simulink model "simulink_rosbag"  (R2020b)
settings: Solver=VariableStepAuto  StartTime=0.0  StopTime=inf  RelTol=1e-3
model workspace (MAT data in the model file):
  Logfile_Data_Object = robotics.ros.BagSelection
  Logfile_Data_Object.FilePath = 'C:\Users\ONLY-GOD\Documents\MATLAB\Examples\R2019b\rosbag\rosbagdata_1.bag'
  Logfile_Data_Object.StartTime = 1606974195.78
  Logfile_Data_Object.EndTime = 1606974582.7
  Logfile_Data_Object.NumMessages = 16443
  Logfile_Data_Object.AvailableTopics = table
  Logfile_Data_Object.AvailableTopics.data{1} = [966; 3865; 11607; 5]
  Logfile_Data_Object.AvailableTopics.data{2} = categorical
  Logfile_Data_Object.AvailableTopics.data{2}.categoryNames = {'nav_msgs/Odometry'; 'rosgraph_msgs/Log'; 'sensor_msgs/Imu'; 'sensor_msgs/NavSatFix'}
  Logfile_Data_Object.AvailableTopics.data{2}.codes = [4; 1; 3; 2]
  Logfile_Data_Object.AvailableTopics.data{3}{1} = '  uint32 Seq
    |   Time Stamp
    |   char FrameId
    | sensor_msgs/NavSatStatus Status
    |   int8 STATUSNOFIX
    |   int8 STATUSFIX
    |   int8 STATUSSBASFIX
    |   int8 STATUSGBASFIX
    |   int8 Status
    |   uint16 SERVICEGPS
    |   uint16 SERVICEGLONASS
    |   uint16 SERVICECOMPASS
    |   uint16 SERVICEGALILEO
    |   uint16 Service
    | double Latitude
    | double Longitude
    | double Altitude
    | double[9] PositionCovariance
    | uint8 COVARIANCETYPEUNKNOWN
    | uint8 COVARIANCETYPEAPPROXIMATED
    | uint8 COVARIANCETYPEDIAGONALKNOWN
    | uint8 COVARIANCETYPEKNOWN
    | uint8 PositionCovarianceType
    | '
  Logfile_Data_Object.AvailableTopics.data{3}{2} = '  uint32 Seq
    |   Time Stamp
    |   char FrameId
    | char ChildFrameId
    | geometry_msgs/PoseWithCovariance Pose
    |   geometry_msgs/Pose Pose
    |     geometry_msgs/Point Position
    |       double X
    |       double Y
    |       double Z
    |     geometry_msgs/Quaternion Orientation
    |       double X
    |       double Y
    |       double Z
    |       double W
    |   double[36] Covariance
    | geometry_msgs/TwistWithCovariance Twist
    |   geometry_msgs/Twist Twist
    |     geometry_msgs/Vector3 Linear
    |       double X
    |       double Y
    |       double Z
    |     geometry_msgs/Vector3 Angular
    |       double X
    |       double Y
    |       double Z
    |   double[36] Covariance
    | '
  Logfile_Data_Object.AvailableTopics.data{3}{3} = '  uint32 Seq
    |   Time Stamp
    |   char FrameId
    | geometry_msgs/Quaternion Orientation
    |   double X
    |   double Y
    |   double Z
    |   double W
    | double[9] OrientationCovariance
    | geometry_msgs/Vector3 AngularVelocity
    |   double X
    |   double Y
    |   double Z
    | double[9] AngularVelocityCovariance
    | geometry_msgs/Vector3 LinearAcceleration
    |   double X
    |   double Y
    |   double Z
    | double[9] LinearAccelerationCovariance
    | '
  Logfile_Data_Object.AvailableTopics.data{3}{4} = 'int8 INFO
    | int8 WARN
    | int8 ERROR
    | int8 FATAL
    | std_msgs/Header Header
    |   uint32 Seq
    |   Time Stamp
    |   char FrameId
    | int8 Level
    | char Name
    | char Msg
    | char File
    | char Function
    | uint32 Line
    | char[] Topics
    | '
  Logfile_Data_Object.AvailableTopics.ndims = 2
  Logfile_Data_Object.AvailableTopics.nrows = 4
  Logfile_Data_Object.AvailableTopics.rownames = {'/fix'; '/husky_velocity_controller/odom'; '/imu/data'; '/rosout'}
  Logfile_Data_Object.AvailableTopics.nvars = 3
  Logfile_Data_Object.AvailableTopics.varnames = {'NumMessages', 'MessageType', 'MessageDefinition'}
  Logfile_Data_Object.AvailableTopics.props.useVariableNamesOriginal = 0
  Logfile_Data_Object.AvailableTopics.props.useDimensionNamesOriginal = 0
  Logfile_Data_Object.AvailableTopics.props.CustomProps = struct()
  Logfile_Data_Object.AvailableTopics.props.VariableCustomProps = struct()
  Logfile_Data_Object.AvailableTopics.props.versionSavedFrom = 4
  Logfile_Data_Object.AvailableTopics.props.minCompatibleVersion = 1
  Logfile_Data_Object.AvailableTopics.props.incompatibilityMsg = ''
  Logfile_Data_Object.AvailableTopics.props.VersionSavedFrom = 4
  Logfile_Data_Object.AvailableTopics.props.Description = ''
  Logfile_Data_Object.AvailableTopics.props.VariableNamesOriginal = {}
  Logfile_Data_Object.AvailableTopics.props.DimensionNames = {'Row', 'Variables'}
  Logfile_Data_Object.AvailableTopics.props.DimensionNamesOriginal = {}
  Logfile_Data_Object.AvailableTopics.props.UserData = []
  Logfile_Data_Object.AvailableTopics.props.VariableDescriptions = {}
  Logfile_Data_Object.AvailableTopics.props.VariableUnits = {}
  Logfile_Data_Object.AvailableTopics.props.VariableContinuity = {}
  Logfile_Data_Object.MessageList = table
  Logfile_Data_Object.MessageList.data{1} = [1606974195.78 1606974195.78 1606974195.78 1606974195.78 1606974196 1606974196.09 1606974196.09 1606974196.09 1606974196.09 1606974196.12 1606974196.13 1606974196.16 ... (16443 elements, 16443x1)]
  Logfile_Data_Object.MessageList.data{2} = categorical
  Logfile_Data_Object.MessageList.data{2}.categoryNames = {'/fix'; '/husky_velocity_controller/odom'; '/imu/data'; '/rosout'}
  Logfile_Data_Object.MessageList.data{2}.codes = [4 4 4 4 4 3 3 2 3 3 2 3 ... (16443 elements, 16443x1)]
  Logfile_Data_Object.MessageList.data{3} = categorical
  Logfile_Data_Object.MessageList.data{3}.categoryNames = {'sensor_msgs/NavSatFix'; 'nav_msgs/Odometry'; 'sensor_msgs/Imu'; 'rosgraph_msgs/Log'}
  Logfile_Data_Object.MessageList.data{3}.codes = [4 4 4 4 4 3 3 2 3 3 2 3 ... (16443 elements, 16443x1)]
  Logfile_Data_Object.MessageList.data{4} = [5486 5746 6008 6272 7849 10576 10942 14932 11308 15691 16057 16816 ... (16443 elements, 16443x1)]
  Logfile_Data_Object.MessageList.ndims = 2
  Logfile_Data_Object.MessageList.nrows = 16443
  Logfile_Data_Object.MessageList.nvars = 4
  Logfile_Data_Object.MessageList.varnames = {'Time', 'Topic', 'MessageType', 'FileOffset'}
  Logfile_Data_Object.MessageList.props.useVariableNamesOriginal = 0
  Logfile_Data_Object.MessageList.props.useDimensionNamesOriginal = 0
  Logfile_Data_Object.MessageList.props.CustomProps = struct()
  Logfile_Data_Object.MessageList.props.VariableCustomProps = struct()
  Logfile_Data_Object.MessageList.props.versionSavedFrom = 4
  Logfile_Data_Object.MessageList.props.minCompatibleVersion = 1
  Logfile_Data_Object.MessageList.props.incompatibilityMsg = ''
  Logfile_Data_Object.MessageList.props.VersionSavedFrom = 4
  Logfile_Data_Object.MessageList.props.Description = ''
  Logfile_Data_Object.MessageList.props.VariableNamesOriginal = {}
  Logfile_Data_Object.MessageList.props.DimensionNames = {'Row', 'Variables'}
  Logfile_Data_Object.MessageList.props.DimensionNamesOriginal = {}
  Logfile_Data_Object.MessageList.props.UserData = []
  Logfile_Data_Object.MessageList.props.VariableDescriptions = {}
  Logfile_Data_Object.MessageList.props.VariableUnits = {}
  Logfile_Data_Object.MessageList.props.VariableContinuity = {}
  Logfile_Data_Object.TopicTypeMap = containers.Map
  Logfile_Data_Object.TopicTypeMap.serialization.keys = {'/fix', '/husky_velocity_controller/odom', '/imu/data', '/rosout'}
  Logfile_Data_Object.TopicTypeMap.serialization.values = {'sensor_msgs/NavSatFix', 'nav_msgs/Odometry', 'sensor_msgs/Imu', 'rosgraph_msgs/Log'}
  Logfile_Data_Object.TopicTypeMap.serialization.uniformity = 1
  Logfile_Data_Object.TopicTypeMap.serialization.keyType = 'char'
  Logfile_Data_Object.TopicTypeMap.serialization.valueType = 'char'
  Logfile_Data_Object.TopicDefinitionMap = containers.Map
  Logfile_Data_Object.TopicDefinitionMap.serialization.keys = {'/fix', '/husky_velocity_controller/odom', '/imu/data', '/rosout'}
  Logfile_Data_Object.TopicDefinitionMap.serialization.values{1} = '  uint32 Seq
    |   Time Stamp
    |   char FrameId
    | sensor_msgs/NavSatStatus Status
    |   int8 STATUSNOFIX
    |   int8 STATUSFIX
    |   int8 STATUSSBASFIX
    |   int8 STATUSGBASFIX
    |   int8 Status
    |   uint16 SERVICEGPS
    |   uint16 SERVICEGLONASS
    |   uint16 SERVICECOMPASS
    |   uint16 SERVICEGALILEO
    |   uint16 Service
    | double Latitude
    | double Longitude
    | double Altitude
    | double[9] PositionCovariance
    | uint8 COVARIANCETYPEUNKNOWN
    | uint8 COVARIANCETYPEAPPROXIMATED
    | uint8 COVARIANCETYPEDIAGONALKNOWN
    | uint8 COVARIANCETYPEKNOWN
    | uint8 PositionCovarianceType
    | '
  Logfile_Data_Object.TopicDefinitionMap.serialization.values{2} = '  uint32 Seq
    |   Time Stamp
    |   char FrameId
    | char ChildFrameId
    | geometry_msgs/PoseWithCovariance Pose
    |   geometry_msgs/Pose Pose
    |     geometry_msgs/Point Position
    |       double X
    |       double Y
    |       double Z
    |     geometry_msgs/Quaternion Orientation
    |       double X
    |       double Y
    |       double Z
    |       double W
    |   double[36] Covariance
    | geometry_msgs/TwistWithCovariance Twist
    |   geometry_msgs/Twist Twist
    |     geometry_msgs/Vector3 Linear
    |       double X
    |       double Y
    |       double Z
    |     geometry_msgs/Vector3 Angular
    |       double X
    |       double Y
    |       double Z
    |   double[36] Covariance
    | '
  Logfile_Data_Object.TopicDefinitionMap.serialization.values{3} = '  uint32 Seq
    |   Time Stamp
    |   char FrameId
    | geometry_msgs/Quaternion Orientation
    |   double X
    |   double Y
    |   double Z
    |   double W
    | double[9] OrientationCovariance
    | geometry_msgs/Vector3 AngularVelocity
    |   double X
    |   double Y
    |   double Z
    | double[9] AngularVelocityCovariance
    | geometry_msgs/Vector3 LinearAcceleration
    |   double X
    |   double Y
    |   double Z
    | double[9] LinearAccelerationCovariance
    | '
  Logfile_Data_Object.TopicDefinitionMap.serialization.values{4} = 'int8 INFO
    | int8 WARN
    | int8 ERROR
    | int8 FATAL
    | std_msgs/Header Header
    |   uint32 Seq
    |   Time Stamp
    |   char FrameId
    | int8 Level
    | char Name
    | char Msg
    | char File
    | char Function
    | uint32 Line
    | char[] Topics
    | '
  Logfile_Data_Object.TopicDefinitionMap.serialization.uniformity = 1
  Logfile_Data_Object.TopicDefinitionMap.serialization.keyType = 'char'
  Logfile_Data_Object.TopicDefinitionMap.serialization.valueType = 'char'
  Logfile_Data_Object.Parser = robotics.ros.internal.tf.TransformationTreeParser
  Logfile_Path = 'C:\Users\ONLY-GOD\Documents\MATLAB\Examples\R2019b\rosbag\rosbagdata_1.bag'
  Logfile_Playback_Duration = nan
  Logfile_Playback_Offset = 0
libraries: robotlib x2
settings Model: Creator=ONLY-GOD  LastModifiedBy=ONLY-GOD

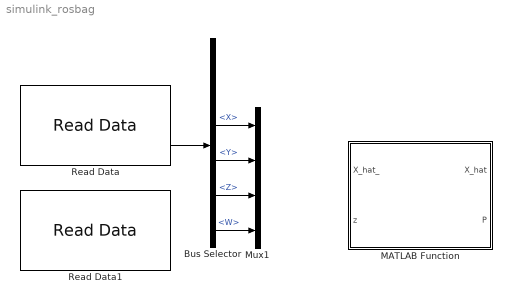
== system simulink_rosbag ==
  Bus Selector : BusSelector  OutputSignals=Pose.Pose.Position.X,Pose.Pose.Position.Y,Pose.Pose.Orientation.X,Pose.Pose.Orientation.Y,Pose.Pose.Orientation.Z,Pose.Pose.Orientation.W
  MATLAB Function : MATLAB Function  TreatAsAtomicUnit=on
  Mux1 : Mux
  Read Data : robotlib/Read Data  topic=/husky_velocity_controller/odom  sampleTime=0.1  logfileType=rosbag  modelName=rostestbag  msgType=nav_msgs/Odometry
      settings: SourceProductBaseCode=RR
  Read Data1 : robotlib/Read Data  topic=/imu/data  sampleTime=0.1  logfileType=rosbag  modelName=rostestbag  msgType=sensor_msgs/Imu
      settings: SourceProductBaseCode=RR
  wires:
  Bus Selector/3 -> Mux1/1  "<X>"
  Bus Selector/4 -> Mux1/2  "<Y>"
  Bus Selector/6 -> Mux1/4  "<W>"
  Bus Selector/5 -> Mux1/3  "<Z>"
  Read Data/2 -> Bus Selector/1

== matlab function simulink_rosbag/MATLAB Function ==
  data: X_hat_ input; X_hat output; z input; P output
function [X_hat,P]=EKF(X_hat_,z)
%State X with the element [x_positin, y_positin, theta_heading, V_linearVelocity, omega_angularVelocity]
x     = X_hat_(1);
y     = X_hat_(2);
theta = X_hat_(3);
V     = X_hat_(4);
omega = X_hat_(5);


%Sampling Time(dt)
dt = 0.01;


%Discretized State Model
X_hat = [x+V*dt*cos(theta);
         y+V*dt*sin(theta);
         theta + omega*dt ;
               V          ;
             omega       ];
         
         
%Jacobian Matrix of the State Transition Matrix F
F = [1 0 -V*dt*sin(theta) dt*cos(theta) 0 ;
     0 1  V*dt*cos(theta) dt*sin(theta) 0 ;
     0 0        1               0       dt;
     0 0        0               1       0 ;
     0 0        0               0       1];
 
%Jacobian Matrix of the Measurement Matrix      H
H=eye(5)*X_hat_;


%Initialization
P = eye(5);

%Prediction Step
X_hat = X_hat;
P     = F*P*F' + Q;

%Update Step
y_tild = z - X_hat;             % measurement residual
K_gain = (P*H')/(H*P*H' + R);
X_hat  = X_hat + K_gain*y_tild;
P      = (eye(5) - K_gain*H)*P;
end
